simulink model "eight_point_dif_2020a"  (R2020a)
settings: Solver=VariableStepAuto  StartTime=0.0  StopTime=10.0  RelTol=1e-3
undefined symbols (not defined in the file): j
settings Model: Creator=eechris  LastModifiedBy=eechris
settings DataIOCC: ReturnWorkspaceOutputs=off
settings DebuggingCC: ArithmeticOperatorsInVariantConditions=warning
settings SFSimCC: SimUseLocalCustomCode=off  CustomCodeUndefinedFunction=UseInterfaceOnly
settings RTWCC: RTWUseLocalCustomCode=off

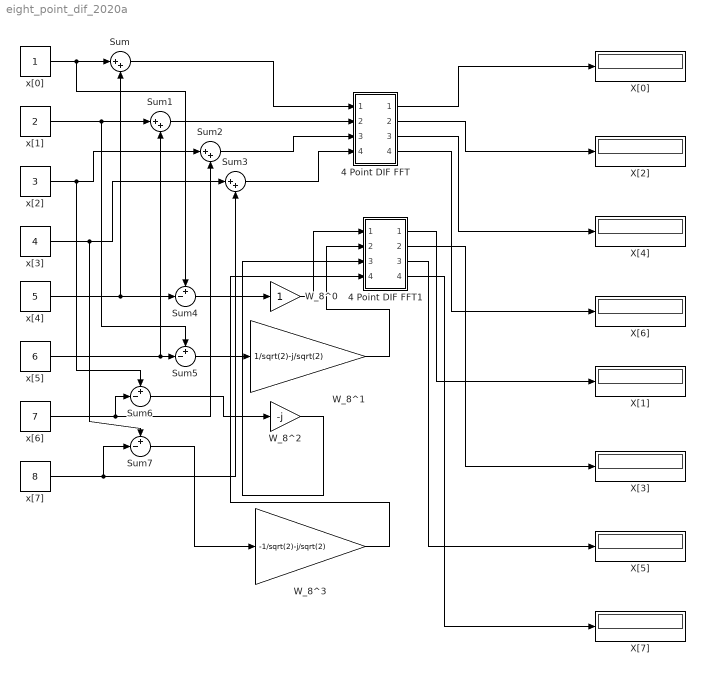
== system eight_point_dif_2020a ==
  4 Point DIF FFT : Subsystem
  4 Point DIF FFT1 : Subsystem
  Sum{,1..3} (4 alike) : Sum  Inputs=|++
  Sum{4..7} (4 alike) : Sum  Inputs=+-|
  W_8^0 : Gain
  W_8^1 : Gain  Gain=1/sqrt(2)-j/sqrt(2)
  W_8^2 : Gain  Gain=-j
  W_8^3 : Gain  Gain=-1/sqrt(2)-j/sqrt(2)
  X[0] : Display
  X[1] : Display
  X[2] : Display
  X[3] : Display
  X[4] : Display
  X[5] : Display
  X[6] : Display
  X[7] : Display
  x[0] : Constant
  x[1] : Constant  Value=2
  x[2] : Constant  Value=3
  x[3] : Constant  Value=4
  x[4] : Constant  Value=5
  x[5] : Constant  Value=6
  x[6] : Constant  Value=7
  x[7] : Constant  Value=8
  wires:
  4 Point DIF FFT/1(Out1) -> X[0]/1
  4 Point DIF FFT/2(Out2) -> X[2]/1
  4 Point DIF FFT/3(Out3) -> X[4]/1
  4 Point DIF FFT/4(Out4) -> X[6]/1
  x[0]/1 -> Sum4/1, Sum/1
  x[4]/1 -> Sum4/2, Sum/2
  Sum/1 -> 4 Point DIF FFT/1(In1)
  Sum1/1 -> 4 Point DIF FFT/2(In2)
  x[1]/1 -> Sum5/1, Sum1/1
  x[5]/1 -> Sum5/2, Sum1/2
  Sum2/1 -> 4 Point DIF FFT/3(In3)
  x[6]/1 -> Sum6/2, Sum2/2
  x[2]/1 -> Sum6/1, Sum2/1
  Sum3/1 -> 4 Point DIF FFT/4(In4)
  x[3]/1 -> Sum7/1, Sum3/1
  x[7]/1 -> Sum7/2, Sum3/2
  Sum7/1 -> W_8^3/1
  Sum6/1 -> W_8^2/1
  Sum5/1 -> W_8^1/1
  Sum4/1 -> W_8^0/1
  W_8^0/1 -> 4 Point DIF FFT1/1(In1)
  W_8^1/1 -> 4 Point DIF FFT1/2(In2)
  W_8^2/1 -> 4 Point DIF FFT1/3(In3)
  W_8^3/1 -> 4 Point DIF FFT1/4(In4)
  4 Point DIF FFT1/4(Out4) -> X[7]/1
  4 Point DIF FFT1/3(Out3) -> X[5]/1
  4 Point DIF FFT1/2(Out2) -> X[3]/1
  4 Point DIF FFT1/1(Out1) -> X[1]/1

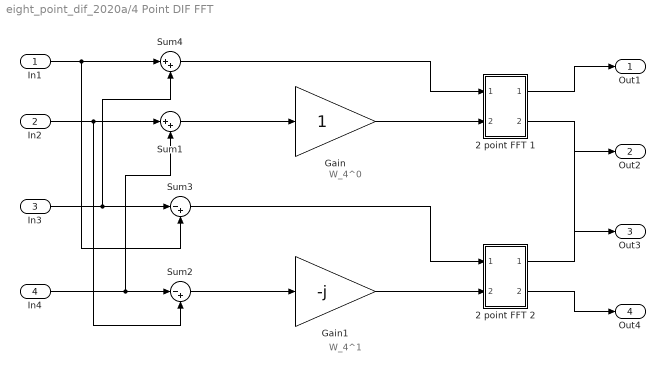
== system eight_point_dif_2020a/4 Point DIF FFT ==
  note: W_4^1
  note: W_4^0
  In1 : Inport
  In2 : Inport  Port=2
  In3 : Inport  Port=3
  In4 : Inport  Port=4
  2 point FFT 1 : Subsystem
  2 point FFT 2 : Subsystem
  Gain : Gain
  Gain1 : Gain  Gain=-j
  Sum1 : Sum  Inputs=|++
  Sum2 : Sum  Inputs=|-+
  Sum3 : Sum  Inputs=|-+
  Sum4 : Sum  Inputs=|++
  Out1 : Outport
  Out2 : Outport  Port=2
  Out3 : Outport  Port=3
  Out4 : Outport  Port=4
  wires:
  2 point FFT 2/1(Out1) -> Out2/1
  Sum2/1 -> Gain1/1
  Sum3/1 -> 2 point FFT 2/1(In1)
  2 point FFT 1/1(Out1) -> Out1/1
  Sum1/1 -> Gain/1
  2 point FFT 1/2(Out2) -> Out3/1
  Gain/1 -> 2 point FFT 1/2(In2)
  In2/1 -> Sum2/2, Sum1/1
  Gain1/1 -> 2 point FFT 2/2(In2)
  2 point FFT 2/2(Out2) -> Out4/1
  Sum4/1 -> 2 point FFT 1/1(In1)
  In4/1 -> Sum1/2, Sum2/1
  In3/1 -> Sum4/2, Sum3/1
  In1/1 -> Sum3/2, Sum4/1

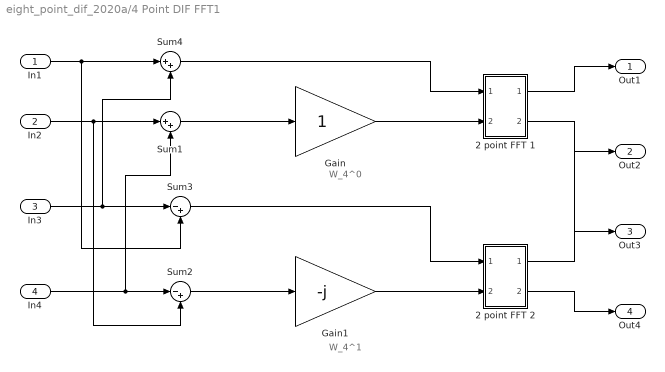
== system eight_point_dif_2020a/4 Point DIF FFT1 ==
  note: W_4^0
  note: W_4^1
  In1 : Inport
  In2 : Inport  Port=2
  In3 : Inport  Port=3
  In4 : Inport  Port=4
  2 point FFT 1 : Subsystem
  2 point FFT 2 : Subsystem
  Gain : Gain
  Gain1 : Gain  Gain=-j
  Sum1 : Sum  Inputs=|++
  Sum2 : Sum  Inputs=|-+
  Sum3 : Sum  Inputs=|-+
  Sum4 : Sum  Inputs=|++
  Out1 : Outport
  Out2 : Outport  Port=2
  Out3 : Outport  Port=3
  Out4 : Outport  Port=4
  wires:
  In1/1 -> Sum4/1, Sum3/2
  In3/1 -> Sum3/1, Sum4/2
  In4/1 -> Sum2/1, Sum1/2
  Sum4/1 -> 2 point FFT 1/1(In1)
  2 point FFT 2/2(Out2) -> Out4/1
  Gain1/1 -> 2 point FFT 2/2(In2)
  In2/1 -> Sum1/1, Sum2/2
  Gain/1 -> 2 point FFT 1/2(In2)
  2 point FFT 1/2(Out2) -> Out3/1
  Sum1/1 -> Gain/1
  2 point FFT 1/1(Out1) -> Out1/1
  Sum3/1 -> 2 point FFT 2/1(In1)
  Sum2/1 -> Gain1/1
  2 point FFT 2/1(Out1) -> Out2/1

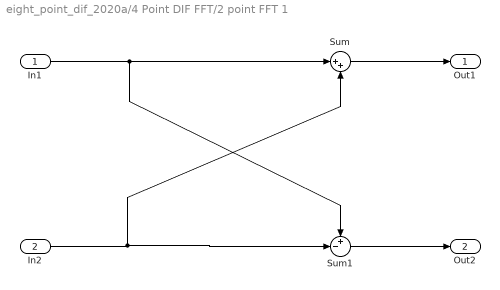
== system eight_point_dif_2020a/4 Point DIF FFT/2 point FFT 1 ==
  In1 : Inport
  In2 : Inport  Port=2
  Sum : Sum  Inputs=|++
  Sum1 : Sum  Inputs=+-|
  Out1 : Outport  VectorParamsAs1DForOutWhenUnconnected=off
  Out2 : Outport  Port=2  VectorParamsAs1DForOutWhenUnconnected=off
  wires:
  Sum/1 -> Out1/1
  In1/1 -> Sum1/1, Sum/1
  Sum1/1 -> Out2/1
  In2/1 -> Sum/2, Sum1/2

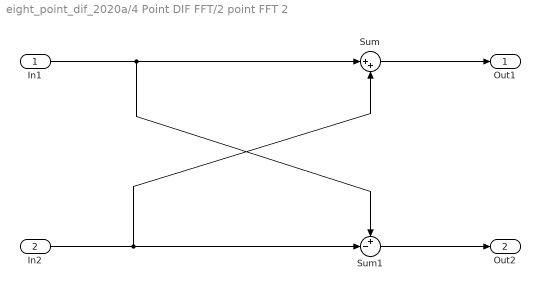
== system eight_point_dif_2020a/4 Point DIF FFT/2 point FFT 2 ==
  In1 : Inport
  In2 : Inport  Port=2
  Sum : Sum  Inputs=|++
  Sum1 : Sum  Inputs=+-|
  Out1 : Outport  VectorParamsAs1DForOutWhenUnconnected=off
  Out2 : Outport  Port=2  VectorParamsAs1DForOutWhenUnconnected=off
  wires:
  In2/1 -> Sum/2, Sum1/2
  Sum1/1 -> Out2/1
  In1/1 -> Sum/1, Sum1/1
  Sum/1 -> Out1/1

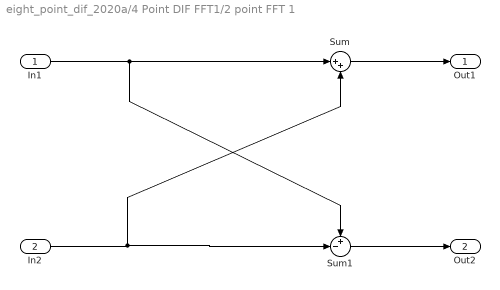
== system eight_point_dif_2020a/4 Point DIF FFT1/2 point FFT 1 ==
  In1 : Inport
  In2 : Inport  Port=2
  Sum : Sum  Inputs=|++
  Sum1 : Sum  Inputs=+-|
  Out1 : Outport  VectorParamsAs1DForOutWhenUnconnected=off
  Out2 : Outport  Port=2  VectorParamsAs1DForOutWhenUnconnected=off
  wires:
  In2/1 -> Sum1/2, Sum/2
  Sum1/1 -> Out2/1
  In1/1 -> Sum/1, Sum1/1
  Sum/1 -> Out1/1

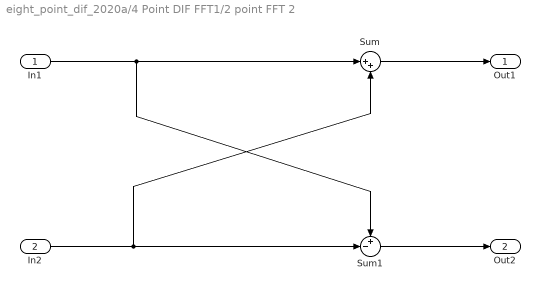
== system eight_point_dif_2020a/4 Point DIF FFT1/2 point FFT 2 ==
  In1 : Inport
  In2 : Inport  Port=2
  Sum : Sum  Inputs=|++
  Sum1 : Sum  Inputs=+-|
  Out1 : Outport  VectorParamsAs1DForOutWhenUnconnected=off
  Out2 : Outport  Port=2  VectorParamsAs1DForOutWhenUnconnected=off
  wires:
  Sum/1 -> Out1/1
  In1/1 -> Sum1/1, Sum/1
  Sum1/1 -> Out2/1
  In2/1 -> Sum1/2, Sum/2
